simulink model "multiple_bus_port_external_RAM"  (Simulink 6.3)
settings: Solver=FixedStepDiscrete  StartTime=0.0  StopTime=10.0  FixedStep=1  RelTol=1e-3
InitFcn:
  | %% DSPBuilder Start
  | alt_dspbuilder_update_model(bdroot)
  | %% DSPBuilder End
undefined symbols (not defined in the file): alt_dspbuilder_update_external_RAM
libraries: alt_dspbuilder_internal_BusSink x2
settings Model: Creator=cpurcell  LastModifiedBy=delphick

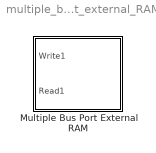
== system multiple_bus_port_external_RAM ==
  Multiple Bus Port External RAM : Subsystem  mask{WRITE_INTERFACES=1, READ_INTERFACES=1, DATA_WIDTH=32, ADDRESS_WIDTH=8, WAIT_STATES_PER_WRITE=0, MAXIMUM_LATENCY=1, SIZE=100, OFFSET=0}
      mask prompts: WRITE_INTERFACES "Number of Write Buses"; READ_INTERFACES "Number of Read Buses"; DATA_WIDTH "Data Width"; ADDRESS_WIDTH "Address Width"; WAIT_STATES_PER_WRITE "Wait States Per Write"; MAXIMUM_LATENCY "Maximum Latency"
      mask help:
      | This is a simulation model of an external RAM block.  It can be used to store and retrieve data from a range of addresses.  It is designed specifically to work with the DSP Builder Video and Image Processing blocks, but may be used for other purposes.
      |
      | As it is a simulation only block, it will not generate HDL when SignalCompiler is run.
      |
      | Parameters
      | =========
      | Data Width - the number of bits used for the data (8,16, 32, 64 or 128 bits only)
      | Address Width - number of bits used for the address (between 1 and 32)
      | Wait States Per Write - choose a fixed number of wait states for each write transfer (between 0 to 10)
      | Maximum Latency - set the latency for pipelined read transfer (between 1 and 255)
      | Size, Offset - to use a range of addresses, choose an offset (start address) and size (number of addresses).  The size added to the offset must be less than 2 ^ address width).
      |
      | Note : If 64 or 128 bits are selected for the data width, the block will attempt to register a Simulink fixed point type of the corresponding width.  This will only work if a valid fixed point license is present on the user's machine.  Please refer to the Simulink help for more information about fixed point licenses.
      mask init:
      | system = gcb;
      | paramNames = get_param(system, 'MaskNames');
      | paramsAndCommas = strcat(paramNames,',');
      | paramValues = eval(['{' paramsAndCommas{:} '}'])';
      | alt_dspbuilder_internal_initMultipleBusPortExternalRAM(system,...
      |             WRITE_INTERFACES, READ_INTERFACES, paramNames, paramValues);
      mask Help: helpview(fullfile(alt_dspbuilder_get_quartus_rootdir, 'dsp_builder', 'docs', 'MultiplePortExternalRAM.html'))

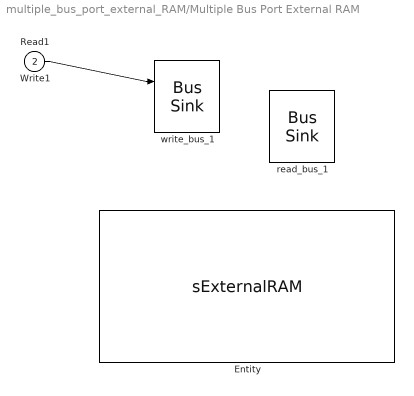
== system multiple_bus_port_external_RAM/Multiple Bus Port External RAM ==
  Write1 : Inport
  Read1 : Inport  Port=2
  Entity : S-Function  InitFcn=alt_dspbuilder_update_external_RAM();  StartFcn=alt_dspbuilder_internal_externalRAMWarning  FunctionName=sExternalRAM  Parameters=WRITE_INTERFACES READ_INTERFACES DATA_WIDTH ADDRESS_WIDTH WAIT_STATES_PER_WRITE MAXIMUM_LATENCY SIZE OFFSET  mask{WRITE_INTERFACES=1, READ_INTERFACES=1, DATA_WIDTH=32, ADDRESS_WIDTH=8, WAIT_STATES_PER_WRITE=0, MAXIMUM_LATENCY=1, SIZE=100, OFFSET=0}
      mask prompts: WRITE_INTERFACES "Number of Write Interfaces"; READ_INTERFACES "Number of Read Interfaces"; DATA_WIDTH "Data Width"; ADDRESS_WIDTH "Address Width"; WAIT_STATES_PER_WRITE "Wait States Per Write"; MAXIMUM_LATENCY "Maximum Latency"
      mask help:
      | This is a simulation model of an external RAM block.  It can be used to store and retrieve data from a range of addresses.  It is designed specifically to work with the DSP Builder Video and Image Processing blocks, but may be used for other purposes.
      |
      | As it is a simulation only block, it will not generate HDL when SignalCompiler is run.
      |
      | Parameters
      | =========
      | Data Width - the number of bits used for the data (8,16, 32, 64 or 128 bits only)
      | Address Width - number of bits used for the address (between 1 and 32)
      | Wait States Per Write - choose a fixed number of wait states for each write transfer (between 0 to 10)
      | Maximum Latency - set the latency for pipelined read transfer (between 1 and 255)
      | Size, Offset - to use a range of addresses, choose an offset (start address) and size (number of addresses).  The size added to the offset must be less than 2 ^ address width).
      |
      | Note : If 64 or 128 bits are selected for the data width, the block will attempt to register a Simulink fixed point type of the corresponding width.  This will only work if a valid fixed point license is present on the user's machine.  Please refer to the Simulink help for more information about fixed point licenses.
      mask Display:
      | port_label('input', 1, 'WriteData1');
      | port_label('input', 2, 'WriteAddress1');
      | port_label('input', 3, 'WriteEnable1');
      | port_label('output', 1, 'WriteWaitRequest1');
      | port_label('input', 4, 'WriteData2');
      | port_label('input', 5, 'WriteAddress2');
      | port_label('input', 6, 'WriteEnable2');
      | port_label('output', 2, 'WriteWaitRequest2');
      | port_label('input', 7, 'WriteData3');
      | port_label('input', 8, 'WriteAddress3');
      | port_label('input', 9, 'WriteEnable3');
      | port_label('output', 3, 'WriteWaitRequest3');
      | port_label('input', 10, 'ReadAddress1');
      | port_label('input', 11, 'ReadEnable1');
      | port_label('output', 4, 'ReadData1');
      | port_label('output', 5, 'ReadDataValid1');
      | port_label('output', 6, 'ReadWaitRequest1');
      | port_label('input', 12, 'ReadAddress2');
      | port_label('input', 13, 'ReadEnable2');
      | port_label('output', 7, 'ReadData2');
      | port_label('output', 8, 'ReadDataValid2');
      | port_label('output', 9, 'ReadWaitRequest2');
  read_bus_1 : alt_dspbuilder_internal_BusSink/Bus Sink  sources={'readdata', 'readdatavalid', 'waitrequest'}  sinks={'address', 'read'}  busType=Memory
  write_bus_1 : alt_dspbuilder_internal_BusSink/Bus Sink  sources={'waitrequest'}  sinks={'writedata','address', 'write'}  busType=Memory
  wires:
  Write1/1 -> write_bus_1/1
